simulink model "Red_problema1_imc_nuevo"  (R2021a)
settings: Solver=ode15s  StartTime=0.0  StopTime=500  MinStep=2e-4  RelTol=1e-3
values from neighbouring files (symbols this model uses):
  area1 = 35.35580060269119    (= 35.3558006027)    [INI.m]    (also in INI_identify.m)
  area1_ini = 34.71685026942442    (= 34.7168502694)    [INI.m]    (also in INI_identify.m)
  area2 = 44.26996515041091    (= 44.2699651504)    [INI.m]    (also in INI_identify.m)
  area2_ini = 42.266246191143715    (= 42.2662461911)    [INI.m]    (also in INI_identify.m)
  area3 = 23.697558590692203    (= 23.6975585907)    [INI.m]    (also in INI_identify.m)
  area3_ini = 22.769214035906693    (= 22.7692140359)    [INI.m]    (also in INI_identify.m)
  area4 = 2.513764303269934    (= 2.51376430327)    [INI.m]    (also in INI_identify.m)
  area4_ini = 2.513764303269934    (= 2.51376430327)    [INI.m]    (also in INI_identify.m)
  area_time = 0    [INI.m]    (also in INI_identify.m)
  bypass_time = 50    [INI.m]    (also in INI_identify.m)
  d_time = 50    [INI.m]    (also in INI_identify.m)
  fcin1 = 0    [INI.m]    (also in INI_identify.m; script_variar_vms.m)
  fcin2 = 0    [INI.m]    (also in INI_identify.m; script_variar_vms.m)
  fcu = 0    [INI.m]    (also in INI_identify.m; script_variar_vms.m)
  fcu_time = 50    [INI.m]    (also in INI_identify.m)
  fhin1 = 0    [INI.m]    (also in INI_identify.m; script_variar_vms.m)
  fhin2 = 0    [INI.m]    (also in INI_identify.m; script_variar_vms.m)
  initials = [uh112_initial uh211_initial uh222_initial uc112_initial uc211_initial uc222_initial fcu_initial]    [INI.m]    (also in INI_identify.m)
  tcin1 = 0    [INI.m]    (also in INI_identify.m; pert_max.m = -5; script_variar_vms.m)
  tcin2 = 0    [INI.m]    (also in INI_identify.m; pert_max.m = -5; script_variar_vms.m)
  thin1 = 0    [INI.m]    (also in INI_identify.m; pert_max.m = 5; script_variar_vms.m)
  thin2 = 0    [INI.m]    (also in INI_identify.m; script_variar_vms.m)
  uc112 = 0.0    (= 0)    [INI.m]    (also in INI_identify.m; script_variar_vms.m)
  uc112_initial = uc112    (= 0)    [INI.m]    (also in INI_identify.m)
  uc211 = 0.0    (= 0)    [INI.m]    (also in INI_identify.m; script_variar_vms.m)
  uc211_initial = uc211    (= 0)    [INI.m]    (also in INI_identify.m)
  uc222 = 0.0    (= 0)    [INI.m]    (also in INI_identify.m; script_variar_vms.m)
  uc222_initial = uc222    (= 0)    [INI.m]    (also in INI_identify.m)
  uh112 = 0.014935258720777856    (= 0.0149352587208)    [INI.m]    (also in INI_identify.m; script_variar_vms.m)
  uh112_initial = uh112    (= 0.0149352587208)    [INI.m]    (also in INI_identify.m)
  uh211 = 0.05299733469368127    (= 0.0529973346937)    [INI.m]    (also in INI_identify.m; script_variar_vms.m)
  uh211_initial = uh211    (= 0.0529973346937)    [INI.m]    (also in INI_identify.m)
  uh222 = 0.08194236649754925    (= 0.0819423664975)    [INI.m]    (also in INI_identify.m; script_variar_vms.m)
  uh222_initial = uh222    (= 0.0819423664975)    [INI.m]    (also in INI_identify.m)
libraries: simulink x4, cstblocks x2
settings Model: Creator=fzpat  LastModifiedBy=LENOVO_T14
settings DataIOCC: SaveFinalState=on  SaveFormat=Array  SaveState=on
settings DebuggingCC: AlgebraicLoopMsg=none  ArtificialAlgebraicLoopMsg=none

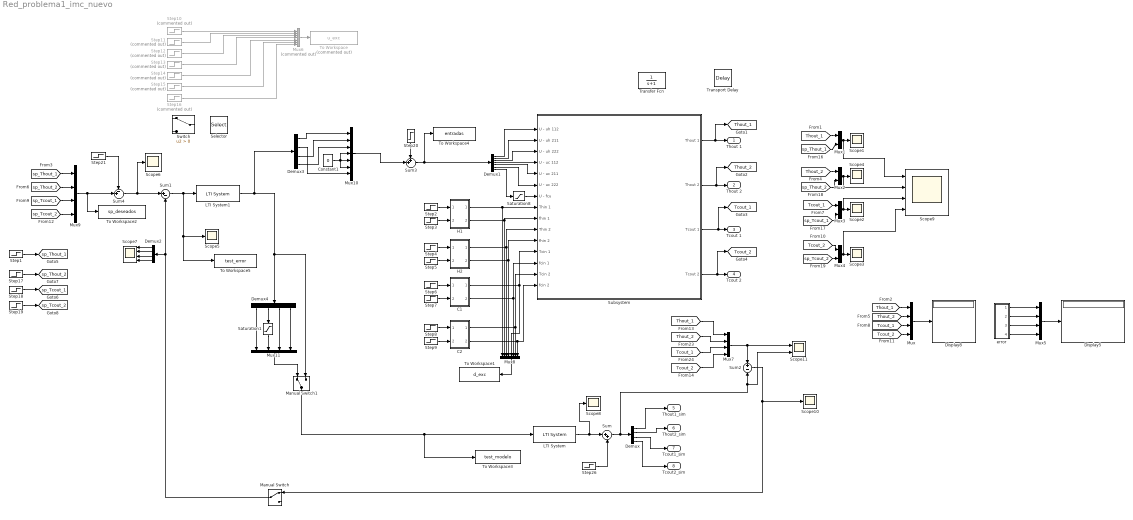
== system Red_problema1_imc_nuevo ==
  C1 : Subsystem
  "C2 " : Subsystem
  Constant1 : Constant  Value=0
  Demux{,2..4} (4 alike) : Demux
  Demux1 : Demux  Outputs=7
  Display5 : Display
  Display8 : Display
  "H1 " : Subsystem
  H2 : Subsystem
  LTI System : cstblocks/LTI System  sys=Gvn1  IC=[]
  LTI System1 : cstblocks/LTI System  sys=Kimc1  IC=[]
  Manual Switch : ManualSwitch
  Manual Switch1 : ManualSwitch
  Mux{,5,7,9,11} (5 alike) : Mux
  Mux{1..4} (4 alike) : Mux  Inputs=2
  Mux10 : Mux  Inputs=7
  Mux6 : Mux  Commented=on  Inputs=7
  Mux8 : Mux  Inputs=8
  Saturation1 : Saturate  UpperLimit=-1e-9  LowerLimit=-29.95
  Saturation8 : Saturate  UpperLimit=-1e-9  LowerLimit=-29.95
  Scope{1..6,8,10} (8 alike) : Scope
  Scope11 : Scope  NumInputPorts=2
  Scope7 : Scope  NumInputPorts=4
  Scope9 : Scope  NumInputPorts=4
  Selector : Selector  InputPortWidth=3  IndexOptions=Index vector (port)  Indices=[1 3]  OutputSizes=1
  Step1 : Step  Time=1e9  Before=385  After=385
  Step10 : Step  Commented=on  Time=bypass_time  Before=uh112_initial  After=uh112
  Step11 : Step  Commented=on  Time=bypass_time  Before=uh211_initial  After=uh211
  Step12 : Step  Commented=on  Time=bypass_time  Before=uh222_initial  After=uh222
  Step13 : Step  Commented=on  Time=bypass_time  Before=uc112_initial  After=uc112
  Step14 : Step  Commented=on  Time=bypass_time  Before=uc211_initial  After=uc211
  Step15 : Step  Commented=on  Time=bypass_time  Before=uc222_initial  After=uc222
  Step16 : Step  Commented=on  Time=fcu_time  After=fcu
  Step17 : Step  Time=1e10  Before=400  After=400
  Step18 : Step  Time=1e9  Before=560  After=560
  Step19 : Step  Time=1e10  Before=340  After=340
  Step2 : Step  Time=d_time  After=thin1
  Step20 : Step  Time=0  Before=initials  After=initials
  Step21 : Step  Time=0  Before=setpoints'  After=setpoints'
  Step26 : Step  Time=0  Before=setpoints'  After=setpoints'
  Step3 : Step  Time=d_time  After=fhin1
  Step4 : Step  Time=d_time  After=thin2
  Step5 : Step  Time=d_time  After=fhin2
  Step6 : Step  Time=d_time  After=tcin1
  Step7 : Step  Time=d_time  After=fcin1
  Step8 : Step  Time=d_time  After=tcin2
  Step9 : Step  Time=d_time  After=fcin2
  Subsystem : Subsystem  TreatAsAtomicUnit=on
      settings: MinAlgLoopOccurrences=on
  Sum : Sum  Inputs=|++
  Sum1 : Sum  Inputs=|+-
  Sum2 : Sum  Inputs=+-
  Sum3 : Sum  Inputs=++|
  Sum4 : Sum  Inputs=-+|
  Switch : Switch  Criteria=u2 > Threshold
  To Workspace : ToWorkspace  Commented=on  VariableName=u_exc  SampleTime=-1
  To Workspace1 : ToWorkspace  VariableName=d_exc  SampleTime=-1
  To Workspace2 : ToWorkspace  VariableName=sp_deseados  SampleTime=-1
  To Workspace3 : ToWorkspace  VariableName=test_modelo  SampleTime=-1
  To Workspace4 : ToWorkspace  VariableName=entradas  SampleTime=-1
  To Workspace5 : ToWorkspace  VariableName=test_error  SampleTime=-1
  Transfer Fcn : TransferFcn  Denominator=[1 1]
  Transport Delay : TransportDelay
  error : Subsystem
  Thout 1 : Outport  VectorParamsAs1DForOutWhenUnconnected=off
  Thout 2 : Outport  Port=2  VectorParamsAs1DForOutWhenUnconnected=off
  Tcout 1 : Outport  Port=3  VectorParamsAs1DForOutWhenUnconnected=off
  Tcout 2 : Outport  Port=4  VectorParamsAs1DForOutWhenUnconnected=off
  Thout1_sim : Outport  Port=5  VectorParamsAs1DForOutWhenUnconnected=off
  Thout2_sim : Outport  Port=6  VectorParamsAs1DForOutWhenUnconnected=off
  Tcout1_sim : Outport  Port=7  VectorParamsAs1DForOutWhenUnconnected=off
  Tcout2_sim : Outport  Port=8  VectorParamsAs1DForOutWhenUnconnected=off
  tag scope: Tcout_1=global, Tcout_2=global, Thout_1=global, Thout_2=global, sp_Tcout_1=global, sp_Tcout_2=global, sp_Thout_1=global, sp_Thout_2=global
  wires:
  Step4/1 -> H2/1(Thin 2)
  Mux5/1 -> Display5/1
  [sp_Tcout_2] -> Mux4/2
  Step16/1 -> Mux6/7
  [Tcout_1] -> Mux/3
  Step15/1 -> Mux6/6
  [Thout_1] -> Mux/1
  error/1(Out1) -> Mux5/1
  [Tcout_1] -> Mux3/1
  Step1/1 -> [sp_Thout_1]
  [Thout_1] -> Mux1/1
  [Tcout_2] -> Mux/4
  Step8/1 -> "C2 "/1(Tcin 2)
  C1/1(Out1) -> Subsystem/12(Tcin 1), Mux8/5
  "C2 "/2(Out2) -> Subsystem/15(fcin 2), Mux8/8
  "C2 "/1(Out1) -> Subsystem/14(Tcin 2), Mux8/7
  C1/2(Out2) -> Subsystem/13(fcin 1), Mux8/6
  Subsystem/4(Tcout 2) -> [Tcout_2], Tcout 2/1
  Step7/1 -> C1/2(fcin 1)
  H2/1(Out1) -> Subsystem/10(Thin 2), Mux8/3
  H2/2(Out2) -> Subsystem/11(fhin 2), Mux8/4
  "H1 "/2(Out2) -> Subsystem/9(fhin 1), Mux8/2
  Step10/1 -> Mux6/1
  Subsystem/1(Thout 1) -> [Thout_1], Thout 1/1
  Step9/1 -> "C2 "/2(fcin 2)
  Subsystem/3(Tcout 1) -> Tcout 1/1, [Tcout_1]
  [Thout_2] -> Mux/2
  LTI System/1 -> Scope8/1, Sum/1
  Step26/1 -> Sum/2
  Demux/2 -> Thout2_sim/1
  "H1 "/1(Out1) -> Mux8/1, Subsystem/8(Thin 1)
  Sum/1 -> Scope11/2, Sum2/2, Demux/1
  Step19/1 -> [sp_Tcout_2]
  Step14/1 -> Mux6/5
  Mux3/1 -> Scope9/3, Scope2/1
  Demux/1 -> Thout1_sim/1
  Step18/1 -> [sp_Tcout_1]
  error/4(Out4) -> Mux5/4
  [Tcout_2] -> Mux4/1
  Mux1/1 -> Scope9/1, Scope1/1
  Demux/4 -> Tcout2_sim/1
  Step13/1 -> Mux6/4
  Demux/3 -> Tcout1_sim/1
  Step12/1 -> Mux6/3
  Step17/1 -> [sp_Thout_2]
  [Thout_2] -> Mux2/1
  Mux2/1 -> Scope9/2, Scope4/1
  Mux8/1 -> To Workspace1/1
  [sp_Tcout_1] -> Mux3/2
  error/3(Out3) -> Mux5/3
  Step6/1 -> C1/1(Tcin 1)
  [sp_Thout_1] -> Mux1/2
  Mux4/1 -> Scope9/4, Scope3/1
  Step11/1 -> Mux6/2
  [sp_Thout_2] -> Mux2/2
  Mux6/1 -> To Workspace/1
  Subsystem/2(Thout 2) -> [Thout_2], Thout 2/1
  error/2(Out2) -> Mux5/2
  Step5/1 -> H2/2(fhin 2)
  Mux/1 -> Display8/1
  Step3/1 -> "H1 "/2(fhin 1)
  Demux1/1 -> Subsystem/1(U - uh 112)
  Demux1/2 -> Subsystem/2(U - uh 211)
  Demux1/3 -> Subsystem/3(U - uh 222)
  Demux1/4 -> Subsystem/4(U - uc 112)
  Demux1/5 -> Subsystem/5(U - uc 211)
  Demux1/6 -> Subsystem/6(U - uc 222)
  [sp_Thout_1] -> Mux9/1
  [sp_Thout_2] -> Mux9/2
  [sp_Tcout_2] -> Mux9/4
  [sp_Tcout_1] -> Mux9/3
  Mux9/1 -> Sum4/2, To Workspace2/1
  Sum1/1 -> To Workspace5/1, Scope5/1, LTI System1/1
  Mux7/1 -> Sum2/1, Scope11/1
  [Thout_1] -> Mux7/1
  [Thout_2] -> Mux7/2
  [Tcout_1] -> Mux7/3
  [Tcout_2] -> Mux7/4
  Demux1/7 -> Saturation8/1
  Sum3/1 -> Demux1/1, To Workspace4/1
  Manual Switch/1 -> Demux2/1, Sum1/2
  LTI System1/1 -> Manual Switch1/2, Demux4/1, Demux3/1
  Sum2/1 -> Manual Switch/1, Scope10/1
  Demux2/1 -> Scope7/1
  Demux2/2 -> Scope7/2
  Demux2/3 -> Scope7/3
  Demux2/4 -> Scope7/4
  Demux3/1 -> Mux10/1
  Demux3/2 -> Mux10/7
  Demux3/3 -> Mux10/2
  Demux3/4 -> Mux10/3
  Constant1/1 -> Mux10/6, Mux10/4, Mux10/5
  Step21/1 -> Sum4/1
  Sum4/1 -> Scope6/1, Sum1/1
  Step20/1 -> Sum3/1
  Mux10/1 -> Sum3/2
  Step2/1 -> "H1 "/1(Thin 1)
  Saturation8/1 -> Subsystem/7(U - fcu)
  Mux11/1 -> Manual Switch1/1
  Demux4/2 -> Saturation1/1
  Saturation1/1 -> Mux11/2
  Demux4/1 -> Mux11/1
  Demux4/3 -> Mux11/3
  Demux4/4 -> Mux11/4
  Manual Switch1/1 -> LTI System/1, To Workspace3/1

== system Red_problema1_imc_nuevo/C1 ==
  Tcin 1 : Inport
  fcin 1 : Inport  Port=2
  Add2 : Sum
  Add3 : Sum
  Constant3 : Constant  Value=300
  Constant4 : Constant  Value=20
  Out1 : Outport  VectorParamsAs1DForOutWhenUnconnected=off
  Out2 : Outport  Port=2  VectorParamsAs1DForOutWhenUnconnected=off
  wires:
  Constant3/1 -> Add2/1
  Constant4/1 -> Add3/1
  Tcin 1/1 -> Add2/2
  fcin 1/1 -> Add3/2
  Add2/1 -> Out1/1
  Add3/1 -> Out2/1

== system Red_problema1_imc_nuevo/C2  ==
  Tcin 2 : Inport
  fcin 2 : Inport  Port=2
  Add4 : Sum
  Add5 : Sum
  Constant5 : Constant  Value=280
  Constant6 : Constant  Value=30
  Out1 : Outport  VectorParamsAs1DForOutWhenUnconnected=off
  Out2 : Outport  Port=2  VectorParamsAs1DForOutWhenUnconnected=off
  wires:
  Constant5/1 -> Add4/1
  Constant6/1 -> Add5/1
  Tcin 2/1 -> Add4/2
  fcin 2/1 -> Add5/2
  Add4/1 -> Out1/1
  Add5/1 -> Out2/1

== system Red_problema1_imc_nuevo/H1  ==
  Thin 1 : Inport
  fhin 1 : Inport  Port=2
  Add : Sum
  Add1 : Sum
  Constant1 : Constant  Value=620
  Constant2 : Constant  Value=10
  Out1 : Outport  VectorParamsAs1DForOutWhenUnconnected=off
  Out2 : Outport  Port=2  VectorParamsAs1DForOutWhenUnconnected=off
  wires:
  Constant1/1 -> Add/1
  Thin 1/1 -> Add/2
  Add/1 -> Out1/1
  Constant2/1 -> Add1/1
  fhin 1/1 -> Add1/2
  Add1/1 -> Out2/1

== system Red_problema1_imc_nuevo/H2 ==
  Thin 2 : Inport
  fhin 2 : Inport  Port=2
  Add : Sum
  Add1 : Sum
  Constant1 : Constant  Value=720
  Constant2 : Constant  Value=15
  Out1 : Outport  VectorParamsAs1DForOutWhenUnconnected=off
  Out2 : Outport  Port=2  VectorParamsAs1DForOutWhenUnconnected=off
  wires:
  Constant1/1 -> Add/1
  Thin 2/1 -> Add/2
  Add/1 -> Out1/1
  Constant2/1 -> Add1/1
  fhin 2/1 -> Add1/2
  Add1/1 -> Out2/1

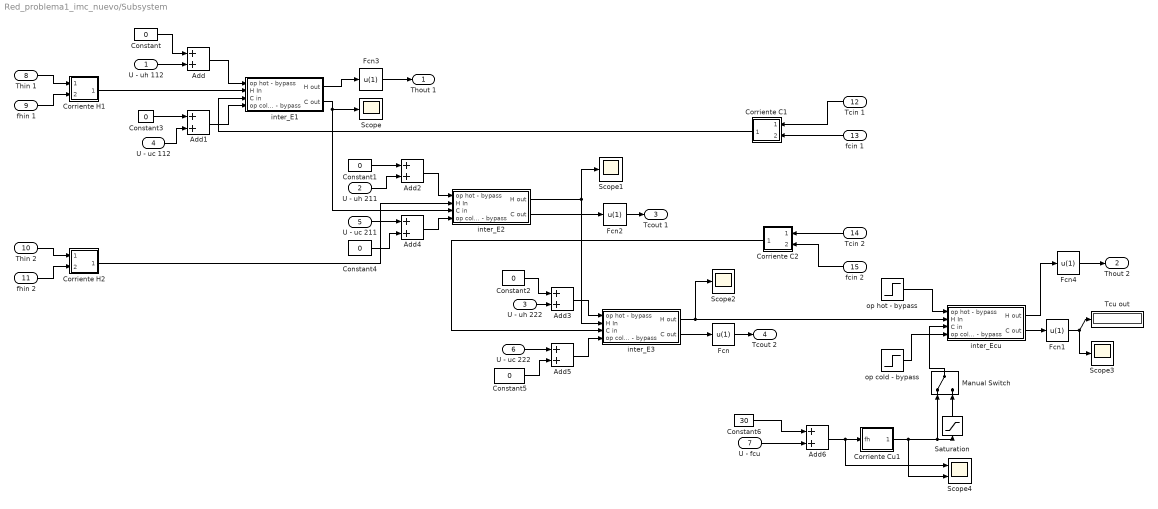
== system Red_problema1_imc_nuevo/Subsystem ==
  U - uh 112 : Inport
  U - uh 211 : Inport  Port=2
  U - uh 222 : Inport  Port=3
  U - uc 112 : Inport  Port=4
  U - uc 211 : Inport  Port=5
  U - uc 222 : Inport  Port=6
  U - fcu : Inport  Port=7
  Thin 1 : Inport  Port=8
  fhin 1 : Inport  Port=9
  Thin 2 : Inport  Port=10
  fhin 2 : Inport  Port=11
  Tcin 1 : Inport  Port=12
  fcin 1 : Inport  Port=13
  Tcin 2 : Inport  Port=14
  fcin 2 : Inport  Port=15
  Add{,1..6} (7 alike) : Sum
  Constant{,1..5} (6 alike) : Constant  Value=0
  Constant6 : Constant  Value=30
  Corriente C1 : Subsystem
  Corriente C2 : Subsystem
  Corriente Cu1 : Subsystem
  Corriente H1 : Subsystem
  Corriente H2 : Subsystem
  Fcn{,1..4} (5 alike) : Fcn  Expr=u(1)
  Manual Switch : ManualSwitch
  Saturation : Saturate  UpperLimit=inf  LowerLimit=1e-9
  Scope{,1..3} (4 alike) : Scope
  Scope4 : Scope  NumInputPorts=2
  Tcu out : Display
  inter_E1 : Subsystem
  inter_E2 : Subsystem
  inter_E3 : Subsystem
  inter_Ecu : Subsystem
  op cold - bypass : Step  Time=0  After=0  SampleTime=0
  op hot - bypass : Step  Time=0  After=0  SampleTime=0
  Thout 1 : Outport  VectorParamsAs1DForOutWhenUnconnected=off
  Thout 2 : Outport  Port=2  VectorParamsAs1DForOutWhenUnconnected=off
  Tcout 1 : Outport  Port=3  VectorParamsAs1DForOutWhenUnconnected=off
  Tcout 2 : Outport  Port=4  VectorParamsAs1DForOutWhenUnconnected=off
  wires:
  inter_Ecu/2(C out) -> Fcn1/1
  op cold - bypass/1 -> inter_Ecu/4("op cold - bypass ")
  Corriente Cu1/1(Out1) -> Saturation/1, Manual Switch/1, Scope4/2
  Corriente H1/1(Out1) -> inter_E1/2(H In)
  inter_Ecu/1(H out) -> Fcn4/1
  Fcn1/1 -> Scope3/1, Tcu out/1
  op hot - bypass/1 -> inter_Ecu/1("op hot - bypass ")
  Thin 1/1 -> Corriente H1/1(In1)
  fhin 1/1 -> Corriente H1/2(In2)
  Tcin 1/1 -> Corriente C1/1(In1)
  fcin 1/1 -> Corriente C1/2(In2)
  Tcin 2/1 -> Corriente C2/1(In1)
  fcin 2/1 -> Corriente C2/2(In2)
  U - uh 112/1 -> Add/2
  Constant/1 -> Add/1
  U - uc 112/1 -> Add1/2
  Add1/1 -> inter_E1/4("op cold - bypass ")
  Add/1 -> inter_E1/1("op hot - bypass ")
  U - uh 211/1 -> Add2/2
  Constant1/1 -> Add2/1
  Add2/1 -> inter_E2/1("op hot - bypass ")
  U - uh 222/1 -> Add3/2
  Add3/1 -> inter_E3/1("op hot - bypass ")
  Constant2/1 -> Add3/1
  Constant3/1 -> Add1/1
  U - uc 211/1 -> Add4/1
  Constant4/1 -> Add4/2
  Add4/1 -> inter_E2/4("op cold - bypass ")
  U - uc 222/1 -> Add5/1
  Constant5/1 -> Add5/2
  Add5/1 -> inter_E3/4("op cold - bypass ")
  Add6/1 -> Scope4/1, Corriente Cu1/1(fh)
  Constant6/1 -> Add6/1
  Thin 2/1 -> Corriente H2/1(In1)
  fhin 2/1 -> Corriente H2/2(In2)
  Corriente H2/1(Out1) -> inter_E2/2(H In)
  Corriente C1/1(Out1) -> inter_E1/3(C in)
  inter_E1/1(H out) -> Fcn3/1
  Fcn3/1 -> Thout 1/1
  inter_E1/2(C out) -> inter_E2/3(C in), Scope/1
  Corriente C2/1(Out1) -> inter_E3/3(C in)
  inter_E3/2(C out) -> Fcn/1
  Fcn/1 -> Tcout 2/1
  inter_E2/1(H out) -> Scope1/1, inter_E3/2(H In)
  inter_E3/1(H out) -> Scope2/1, inter_Ecu/2(H In)
  Fcn4/1 -> Thout 2/1
  inter_E2/2(C out) -> Fcn2/1
  Fcn2/1 -> Tcout 1/1
  U - fcu/1 -> Add6/2
  Saturation/1 -> Manual Switch/2
  Manual Switch/1 -> inter_Ecu/3(C in)

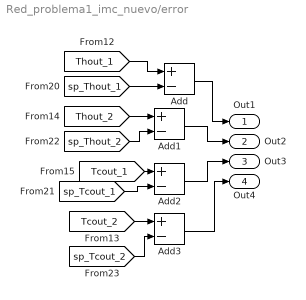
== system Red_problema1_imc_nuevo/error ==
  Add{,1..3} (4 alike) : Sum  Inputs=+-
  Out1 : Outport  VectorParamsAs1DForOutWhenUnconnected=off
  Out2 : Outport  Port=2  VectorParamsAs1DForOutWhenUnconnected=off
  Out3 : Outport  Port=3  VectorParamsAs1DForOutWhenUnconnected=off
  Out4 : Outport  Port=4  VectorParamsAs1DForOutWhenUnconnected=off
  wires:
  [sp_Thout_2] -> Add1/2
  [sp_Tcout_2] -> Add3/2
  [sp_Tcout_1] -> Add2/2
  [sp_Thout_1] -> Add/2
  [Thout_2] -> Add1/1
  [Thout_1] -> Add/1
  [Tcout_1] -> Add2/1
  [Tcout_2] -> Add3/1
  Add1/1 -> Out2/1
  Add/1 -> Out1/1
  Add3/1 -> Out4/1
  Add2/1 -> Out3/1

== system Red_problema1_imc_nuevo/Subsystem/Corriente C1 ==
  In1 : Inport
  In2 : Inport  Port=2
  Mux5 : Mux  Inputs=3
  Terminator : Terminator
  Terminator1 : Terminator
  fc : Step  Before=13  After=13  SampleTime=0
  hc : Step  Before=1  SampleTime=0
  tc : Step  Before=333  After=333  SampleTime=0
  Out1 : Outport  VectorParamsAs1DForOutWhenUnconnected=off
  wires:
  Mux5/1 -> Out1/1
  hc/1 -> Mux5/3
  In1/1 -> Mux5/1
  In2/1 -> Mux5/2
  fc/1 -> Terminator/1
  tc/1 -> Terminator1/1

== system Red_problema1_imc_nuevo/Subsystem/Corriente C2 ==
  In1 : Inport
  In2 : Inport  Port=2
  Mux5 : Mux  Inputs=3
  Terminator : Terminator
  Terminator1 : Terminator
  fh : Step  Before=12  After=12  SampleTime=0
  hh : Step  Before=1  SampleTime=0
  th : Step  Time=2  Before=293  After=293  SampleTime=0
  Out1 : Outport  VectorParamsAs1DForOutWhenUnconnected=off
  wires:
  hh/1 -> Mux5/3
  Mux5/1 -> Out1/1
  In1/1 -> Mux5/1
  In2/1 -> Mux5/2
  fh/1 -> Terminator/1
  th/1 -> Terminator1/1

== system Red_problema1_imc_nuevo/Subsystem/Corriente Cu1 ==
  fh : Inport
  Mux5 : Mux  Inputs=3
  hh : Step  Before=1  SampleTime=0
  th : Step  Time=2  Before=283  After=283  SampleTime=0
  Out1 : Outport  VectorParamsAs1DForOutWhenUnconnected=off
  wires:
  hh/1 -> Mux5/3
  th/1 -> Mux5/1
  Mux5/1 -> Out1/1
  fh/1 -> Mux5/2

== system Red_problema1_imc_nuevo/Subsystem/Corriente H1 ==
  In1 : Inport
  In2 : Inport  Port=2
  Mux5 : Mux  Inputs=3
  Terminator : Terminator
  Terminator1 : Terminator
  fh : Step  Before=20  After=20  SampleTime=0
  hh : Step  Before=1  SampleTime=0
  th : Step  Time=2  Before=423  After=423  SampleTime=0
  Out1 : Outport  VectorParamsAs1DForOutWhenUnconnected=off
  wires:
  Mux5/1 -> Out1/1
  hh/1 -> Mux5/3
  In1/1 -> Mux5/1
  In2/1 -> Mux5/2
  th/1 -> Terminator/1
  fh/1 -> Terminator1/1

== system Red_problema1_imc_nuevo/Subsystem/Corriente H2 ==
  In1 : Inport
  In2 : Inport  Port=2
  Mux5 : Mux  Inputs=3
  Terminator : Terminator
  Terminator1 : Terminator
  fh : Step  Before=20  After=20  SampleTime=0
  hh : Step  Before=1  SampleTime=0
  th : Step  Time=2  Before=423  After=423  SampleTime=0
  Out1 : Outport  VectorParamsAs1DForOutWhenUnconnected=off
  wires:
  Mux5/1 -> Out1/1
  hh/1 -> Mux5/3
  In1/1 -> Mux5/1
  In2/1 -> Mux5/2
  th/1 -> Terminator/1
  fh/1 -> Terminator1/1

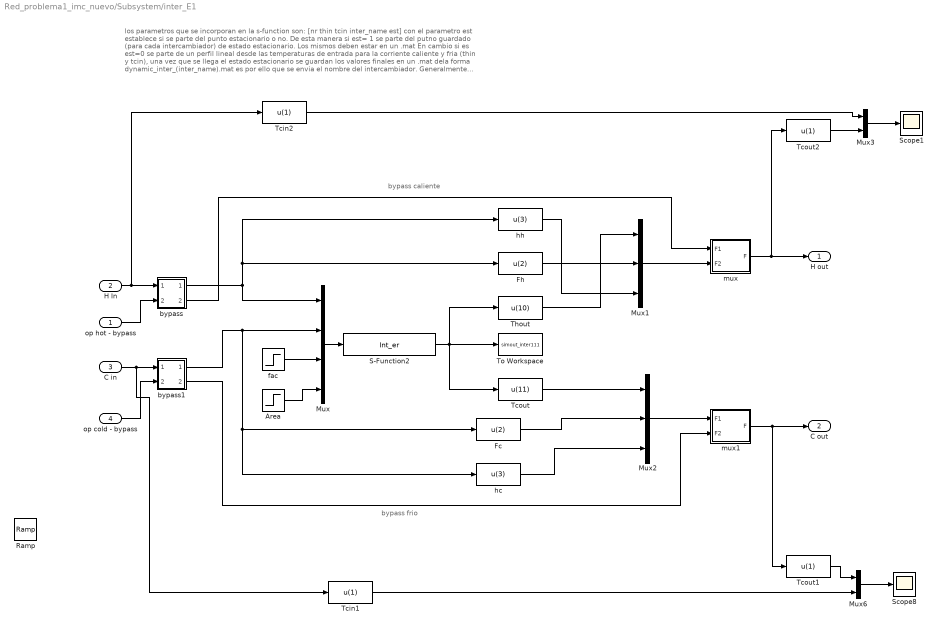
== system Red_problema1_imc_nuevo/Subsystem/inter_E1 ==
  note: los parametros que se incorporan en la s-function son: [nr thin tcin inter_name est]
      | con el parametro est establece si se parte del punto estacionario o no. De esta manera si est= 1 se parte del putno guardado (para cada intercambiador) de estado estacionario. Los mismos deben estar en un .mat
      | En cambio si es est=0 se parte de un perfil lineal  desde las temperaturas de entrada para la corriente caliente y fria (thin y tcin), una vez que se llega el estado estacionario se guardan los valores finales en un .mat
      | dela forma dynamic_inter_(inter_name).mat   es por ello que se envia el nombre del intercambiador.
      | Generalmente para la primera vez que se corre la red se una est=0 para que llegue al estado estacionario y una vez que se alcanzó se vuelve a correr con est= 1 para hacer análisis de control
  note: bypass frio
  note: bypass caliente
  "op hot - bypass " : Inport
  H In : Inport  Port=2
  C in : Inport  Port=3
  "op cold - bypass " : Inport  Port=4
  Area : Step  Time=area_time  Before=area1_ini  After=area1  SampleTime=0
  Fc : Fcn  Expr=u(2)
  Fh : Fcn  Expr=u(2)
  Mux : Mux
  Mux1 : Mux  Inputs=3
  Mux2 : Mux  Inputs=3
  Mux3 : Mux  Inputs=2
  Mux6 : Mux  Inputs=2
  Ramp : simulink/Sources/Ramp  slope=0  start=0  InitialOutput=0
  S-Function2 : S-Function  FunctionName=Int_er  Parameters=10 620 300 112 2  SFunctionDeploymentMode=off  EnableBusSupport=off
  Scope1 : Scope
  Scope8 : Scope
  Tcin1 : Fcn  Expr=u(1)
  Tcin2 : Fcn  Expr=u(1)
  Tcout : Fcn  Expr=u(11)
  Tcout1 : Fcn  Expr=u(1)
  Tcout2 : Fcn  Expr=u(1)
  Thout : Fcn  Expr=u(10)
  To Workspace : ToWorkspace  VariableName=simout_inter111  SampleTime=-1
  bypass : Subsystem
  bypass1 : Subsystem
  fac : Step  After=0  SampleTime=0
  hc : Fcn  Expr=u(3)
  hh : Fcn  Expr=u(3)
  mux : Subsystem
  mux1 : Subsystem
  H out : Outport  VectorParamsAs1DForOutWhenUnconnected=off
  C out : Outport  Port=2  VectorParamsAs1DForOutWhenUnconnected=off
  wires:
  Tcout/1 -> Mux2/1
  Thout/1 -> Mux1/1
  Fc/1 -> Mux2/2
  Fh/1 -> Mux1/2
  S-Function2/1 -> Thout/1, To Workspace/1, Tcout/1
  Mux/1 -> S-Function2/1
  fac/1 -> Mux/3
  hc/1 -> Mux2/3
  hh/1 -> Mux1/3
  Area/1 -> Mux/4
  H In/1 -> Tcin2/1, bypass/1(1)
  bypass/1(" 1") -> Mux/1, Fh/1, hh/1
  Mux1/1 -> mux/2(F2)
  bypass/2(" 2") -> mux/1(F1)
  "op hot - bypass "/1 -> bypass/2(u122)
  C in/1 -> Tcin1/1, bypass1/1(1)
  "op cold - bypass "/1 -> bypass1/2(u122)
  mux/1("F ") -> Tcout2/1, H out/1
  Mux2/1 -> mux1/1(F1)
  mux1/1("F ") -> Tcout1/1, C out/1
  bypass1/1(" 1") -> hc/1, Fc/1, Mux/2
  bypass1/2(" 2") -> mux1/2(F2)
  Mux6/1 -> Scope8/1
  Tcout1/1 -> Mux6/1
  Tcin1/1 -> Mux6/2
  Mux3/1 -> Scope1/1
  Tcout2/1 -> Mux3/2
  Tcin2/1 -> Mux3/1

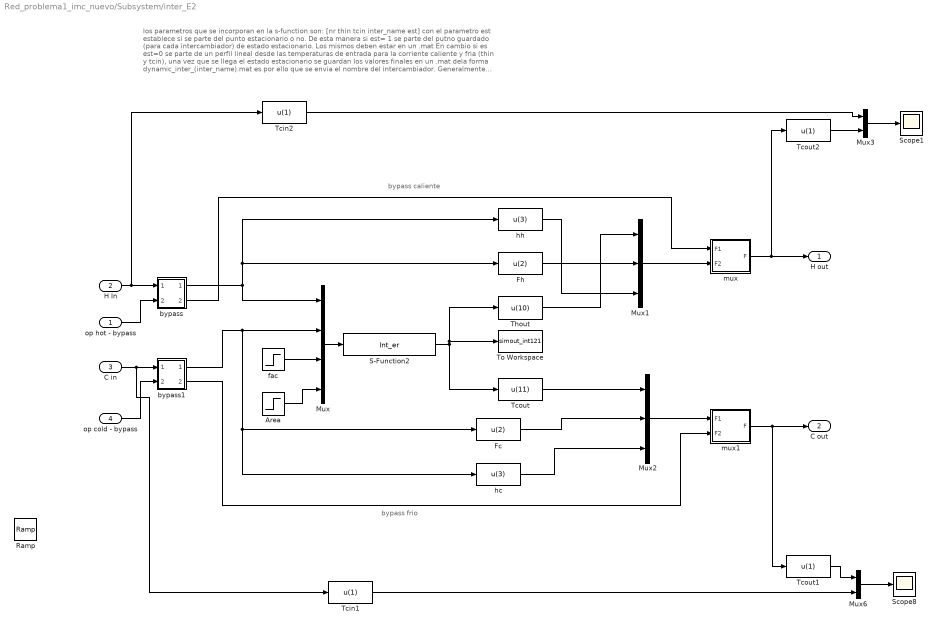
== system Red_problema1_imc_nuevo/Subsystem/inter_E2 ==
  note: bypass caliente
  note: bypass frio
  note: los parametros que se incorporan en la s-function son: [nr thin tcin inter_name est]
      | con el parametro est establece si se parte del punto estacionario o no. De esta manera si est= 1 se parte del putno guardado (para cada intercambiador) de estado estacionario. Los mismos deben estar en un .mat
      | En cambio si es est=0 se parte de un perfil lineal  desde las temperaturas de entrada para la corriente caliente y fria (thin y tcin), una vez que se llega el estado estacionario se guardan los valores finales en un .mat
      | dela forma dynamic_inter_(inter_name).mat   es por ello que se envia el nombre del intercambiador.
      | Generalmente para la primera vez que se corre la red se una est=0 para que llegue al estado estacionario y una vez que se alcanzó se vuelve a correr con est= 1 para hacer análisis de control
  "op hot - bypass " : Inport
  H In : Inport  Port=2
  C in : Inport  Port=3
  "op cold - bypass " : Inport  Port=4
  Area : Step  Time=area_time  Before=area2_ini  After=area2  SampleTime=0
  Fc : Fcn  Expr=u(2)
  Fh : Fcn  Expr=u(2)
  Mux : Mux
  Mux1 : Mux  Inputs=3
  Mux2 : Mux  Inputs=3
  Mux3 : Mux  Inputs=2
  Mux6 : Mux  Inputs=2
  Ramp : simulink/Sources/Ramp  slope=0  start=0  InitialOutput=0
  S-Function2 : S-Function  FunctionName=Int_er  Parameters=10 720 417.5 211 2  SFunctionDeploymentMode=off  EnableBusSupport=off
  Scope1 : Scope
  Scope8 : Scope
  Tcin1 : Fcn  Expr=u(1)
  Tcin2 : Fcn  Expr=u(1)
  Tcout : Fcn  Expr=u(11)
  Tcout1 : Fcn  Expr=u(1)
  Tcout2 : Fcn  Expr=u(1)
  Thout : Fcn  Expr=u(10)
  To Workspace : ToWorkspace  VariableName=simout_int121  SampleTime=-1
  bypass : Subsystem
  bypass1 : Subsystem
  fac : Step  After=0  SampleTime=0
  hc : Fcn  Expr=u(3)
  hh : Fcn  Expr=u(3)
  mux : Subsystem
  mux1 : Subsystem
  H out : Outport  VectorParamsAs1DForOutWhenUnconnected=off
  C out : Outport  Port=2  VectorParamsAs1DForOutWhenUnconnected=off
  wires:
  Tcin2/1 -> Mux3/1
  Tcout2/1 -> Mux3/2
  Mux3/1 -> Scope1/1
  Tcin1/1 -> Mux6/2
  Tcout1/1 -> Mux6/1
  Mux6/1 -> Scope8/1
  bypass1/2(" 2") -> mux1/2(F2)
  bypass1/1(" 1") -> Mux/2, Fc/1, hc/1
  mux1/1("F ") -> C out/1, Tcout1/1
  Mux2/1 -> mux1/1(F1)
  mux/1("F ") -> H out/1, Tcout2/1
  "op cold - bypass "/1 -> bypass1/2(u122)
  C in/1 -> bypass1/1(1), Tcin1/1
  "op hot - bypass "/1 -> bypass/2(u122)
  bypass/2(" 2") -> mux/1(F1)
  Mux1/1 -> mux/2(F2)
  bypass/1(" 1") -> hh/1, Fh/1, Mux/1
  H In/1 -> bypass/1(1), Tcin2/1
  Area/1 -> Mux/4
  hh/1 -> Mux1/3
  hc/1 -> Mux2/3
  fac/1 -> Mux/3
  Mux/1 -> S-Function2/1
  S-Function2/1 -> Tcout/1, To Workspace/1, Thout/1
  Fh/1 -> Mux1/2
  Fc/1 -> Mux2/2
  Thout/1 -> Mux1/1
  Tcout/1 -> Mux2/1

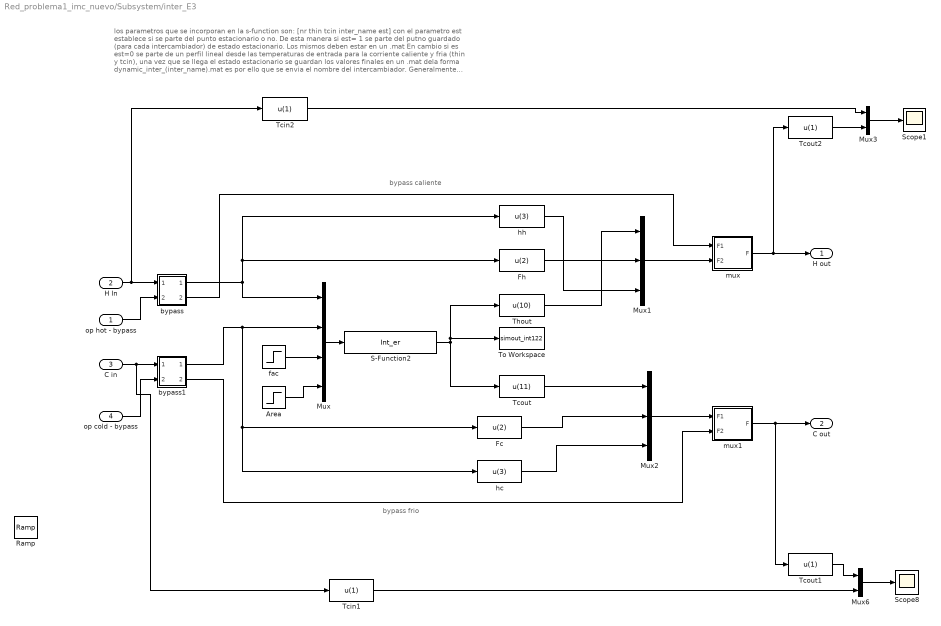
== system Red_problema1_imc_nuevo/Subsystem/inter_E3 ==
  note: bypass frio
  note: bypass caliente
  note: los parametros que se incorporan en la s-function son: [nr thin tcin inter_name est]
      | con el parametro est establece si se parte del punto estacionario o no. De esta manera si est= 1 se parte del putno guardado (para cada intercambiador) de estado estacionario. Los mismos deben estar en un .mat
      | En cambio si es est=0 se parte de un perfil lineal  desde las temperaturas de entrada para la corriente caliente y fria (thin y tcin), una vez que se llega el estado estacionario se guardan los valores finales en un .mat
      | dela forma dynamic_inter_(inter_name).mat   es por ello que se envia el nombre del intercambiador.
      | Generalmente para la primera vez que se corre la red se una est=0 para que llegue al estado estacionario y una vez que se alcanzó se vuelve a correr con est= 1 para hacer análisis de control
  "op hot - bypass " : Inport
  H In : Inport  Port=2
  C in : Inport  Port=3
  "op cold - bypass " : Inport  Port=4
  Area : Step  Time=area_time  Before=area3_ini  After=area3  SampleTime=0
  Fc : Fcn  Expr=u(2)
  Fh : Fcn  Expr=u(2)
  Mux : Mux
  Mux1 : Mux  Inputs=3
  Mux2 : Mux  Inputs=3
  Mux3 : Mux  Inputs=2
  Mux6 : Mux  Inputs=2
  Ramp : simulink/Sources/Ramp  slope=0  start=0  InitialOutput=0
  S-Function2 : S-Function  FunctionName=Int_er  Parameters=10 530 280 222 2  SFunctionDeploymentMode=off  EnableBusSupport=off
  Scope1 : Scope
  Scope8 : Scope
  Tcin1 : Fcn  Expr=u(1)
  Tcin2 : Fcn  Expr=u(1)
  Tcout : Fcn  Expr=u(11)
  Tcout1 : Fcn  Expr=u(1)
  Tcout2 : Fcn  Expr=u(1)
  Thout : Fcn  Expr=u(10)
  To Workspace : ToWorkspace  VariableName=simout_int122  SampleTime=-1
  bypass : Subsystem
  bypass1 : Subsystem
  fac : Step  After=0  SampleTime=0
  hc : Fcn  Expr=u(3)
  hh : Fcn  Expr=u(3)
  mux : Subsystem
  mux1 : Subsystem
  H out : Outport  VectorParamsAs1DForOutWhenUnconnected=off
  C out : Outport  Port=2  VectorParamsAs1DForOutWhenUnconnected=off
  wires:
  Tcout/1 -> Mux2/1
  Thout/1 -> Mux1/1
  Fc/1 -> Mux2/2
  Fh/1 -> Mux1/2
  S-Function2/1 -> Thout/1, To Workspace/1, Tcout/1
  Mux/1 -> S-Function2/1
  fac/1 -> Mux/3
  hc/1 -> Mux2/3
  hh/1 -> Mux1/3
  Area/1 -> Mux/4
  H In/1 -> Tcin2/1, bypass/1(1)
  bypass/1(" 1") -> Mux/1, Fh/1, hh/1
  Mux1/1 -> mux/2(F2)
  bypass/2(" 2") -> mux/1(F1)
  "op hot - bypass "/1 -> bypass/2(u122)
  C in/1 -> Tcin1/1, bypass1/1(1)
  "op cold - bypass "/1 -> bypass1/2(u122)
  mux/1("F ") -> Tcout2/1, H out/1
  Mux2/1 -> mux1/1(F1)
  mux1/1("F ") -> Tcout1/1, C out/1
  bypass1/1(" 1") -> hc/1, Fc/1, Mux/2
  bypass1/2(" 2") -> mux1/2(F2)
  Mux6/1 -> Scope8/1
  Tcout1/1 -> Mux6/1
  Tcin1/1 -> Mux6/2
  Mux3/1 -> Scope1/1
  Tcout2/1 -> Mux3/2
  Tcin2/1 -> Mux3/1

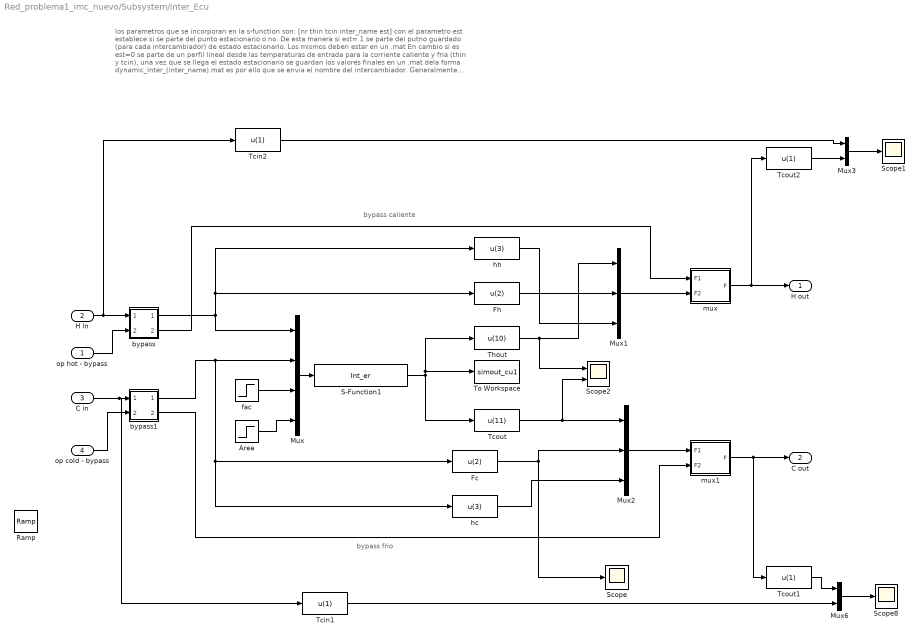
== system Red_problema1_imc_nuevo/Subsystem/inter_Ecu ==
  note: bypass caliente
  note: bypass frio
  note: los parametros que se incorporan en la s-function son: [nr thin tcin inter_name est]
      | con el parametro est establece si se parte del punto estacionario o no. De esta manera si est= 1 se parte del putno guardado (para cada intercambiador) de estado estacionario. Los mismos deben estar en un .mat
      | En cambio si es est=0 se parte de un perfil lineal  desde las temperaturas de entrada para la corriente caliente y fria (thin y tcin), una vez que se llega el estado estacionario se guardan los valores finales en un .mat
      | dela forma dynamic_inter_(inter_name).mat   es por ello que se envia el nombre del intercambiador.
      | Generalmente para la primera vez que se corre la red se una est=0 para que llegue al estado estacionario y una vez que se alcanzó se vuelve a correr con est= 1 para hacer análisis de control
  "op hot - bypass " : Inport
  H In : Inport  Port=2
  C in : Inport  Port=3
  "op cold - bypass " : Inport  Port=4
  Area : Step  Time=area_time  Before=area4_ini  After=area4  SampleTime=0
  Fc : Fcn  Expr=u(2)
  Fh : Fcn  Expr=u(2)
  Mux : Mux
  Mux1 : Mux  Inputs=3
  Mux2 : Mux  Inputs=3
  Mux3 : Mux  Inputs=2
  Mux6 : Mux  Inputs=2
  Ramp : simulink/Sources/Ramp  slope=0.9/150  start=30  InitialOutput=0
  S-Function1 : S-Function  FunctionName=Int_er  Parameters=10 410 293 02 2  SFunctionDeploymentMode=off  EnableBusSupport=off
  Scope : Scope
  Scope1 : Scope
  Scope2 : Scope  NumInputPorts=2
  Scope8 : Scope
  Tcin1 : Fcn  Expr=u(1)
  Tcin2 : Fcn  Expr=u(1)
  Tcout : Fcn  Expr=u(11)
  Tcout1 : Fcn  Expr=u(1)
  Tcout2 : Fcn  Expr=u(1)
  Thout : Fcn  Expr=u(10)
  To Workspace : ToWorkspace  VariableName=simout_cu1  SampleTime=-1
  bypass : Subsystem
  bypass1 : Subsystem
  fac : Step  After=0  SampleTime=0
  hc : Fcn  Expr=u(3)
  hh : Fcn  Expr=u(3)
  mux : Subsystem
  mux1 : Subsystem
  H out : Outport  VectorParamsAs1DForOutWhenUnconnected=off
  C out : Outport  Port=2  VectorParamsAs1DForOutWhenUnconnected=off
  wires:
  Tcin2/1 -> Mux3/1
  Tcout2/1 -> Mux3/2
  Mux3/1 -> Scope1/1
  Tcin1/1 -> Mux6/2
  Tcout1/1 -> Mux6/1
  Mux6/1 -> Scope8/1
  bypass1/2(" 2") -> mux1/2(F2)
  bypass1/1(" 1") -> Mux/2, Fc/1, hc/1
  mux1/1("F ") -> C out/1, Tcout1/1
  Mux2/1 -> mux1/1(F1)
  mux/1("F ") -> H out/1, Tcout2/1
  C in/1 -> bypass1/1(1), Tcin1/1
  "op hot - bypass "/1 -> bypass/2(u122)
  bypass/2(" 2") -> mux/1(F1)
  Mux1/1 -> mux/2(F2)
  bypass/1(" 1") -> hh/1, Fh/1, Mux/1
  H In/1 -> bypass/1(1), Tcin2/1
  Area/1 -> Mux/4
  hh/1 -> Mux1/3
  hc/1 -> Mux2/3
  fac/1 -> Mux/3
  Mux/1 -> S-Function1/1
  S-Function1/1 -> Tcout/1, To Workspace/1, Thout/1
  Fh/1 -> Mux1/2
  Fc/1 -> Mux2/2, Scope/1
  Thout/1 -> Scope2/1, Mux1/1
  Tcout/1 -> Scope2/2, Mux2/1
  "op cold - bypass "/1 -> bypass1/2(u122)

== system Red_problema1_imc_nuevo/Subsystem/inter_E1/bypass ==
  note: la corriete 2 es la corriente del byapass
  note: la corriente 1 es la que se introduce al intercambiador
  1 : Inport
  u122 : Inport  Port=2
  Add : Sum  Inputs=+-
  Manual Switch : ManualSwitch  CurrentSetting=0
  Mux : Mux  Inputs=3
  Mux1 : Mux  Inputs=3
  Product : Product
  Saturation : Saturate  UpperLimit=0.999999999  LowerLimit=0
  T : Fcn  Expr=u(1)
  f : Fcn  Expr=u(2)
  h : Fcn  Expr=u(3)
  " 1" : Outport  VectorParamsAs1DForOutWhenUnconnected=off
  " 2" : Outport  Port=2  VectorParamsAs1DForOutWhenUnconnected=off
  wires:
  f/1 -> Add/1, Product/2
  Product/1 -> Mux1/2, Add/2
  1/1 -> T/1, h/1, f/1
  Add/1 -> Mux/2
  h/1 -> Mux1/3, Mux/3
  T/1 -> Mux1/1, Mux/1
  Mux/1 -> " 1"/1
  Mux1/1 -> " 2"/1
  u122/1 -> Manual Switch/2, Saturation/1
  Saturation/1 -> Manual Switch/1
  Manual Switch/1 -> Product/1

== system Red_problema1_imc_nuevo/Subsystem/inter_E1/bypass1 ==
  note: la corriente 1 es la que se introduce al intercambiador
  note: la corriete 2 es la corriente del byapass
  1 : Inport
  u122 : Inport  Port=2
  Add : Sum  Inputs=+-
  Manual Switch : ManualSwitch  CurrentSetting=0
  Mux : Mux  Inputs=3
  Mux1 : Mux  Inputs=3
  Product : Product
  Saturation : Saturate  UpperLimit=0.999999999  LowerLimit=0
  T : Fcn  Expr=u(1)
  f : Fcn  Expr=u(2)
  h : Fcn  Expr=u(3)
  " 1" : Outport  VectorParamsAs1DForOutWhenUnconnected=off
  " 2" : Outport  Port=2  VectorParamsAs1DForOutWhenUnconnected=off
  wires:
  Mux1/1 -> " 2"/1
  Mux/1 -> " 1"/1
  T/1 -> Mux/1, Mux1/1
  h/1 -> Mux/3, Mux1/3
  Add/1 -> Mux/2
  1/1 -> f/1, h/1, T/1
  Product/1 -> Add/2, Mux1/2
  f/1 -> Product/2, Add/1
  Saturation/1 -> Manual Switch/1
  u122/1 -> Manual Switch/2, Saturation/1
  Manual Switch/1 -> Product/1

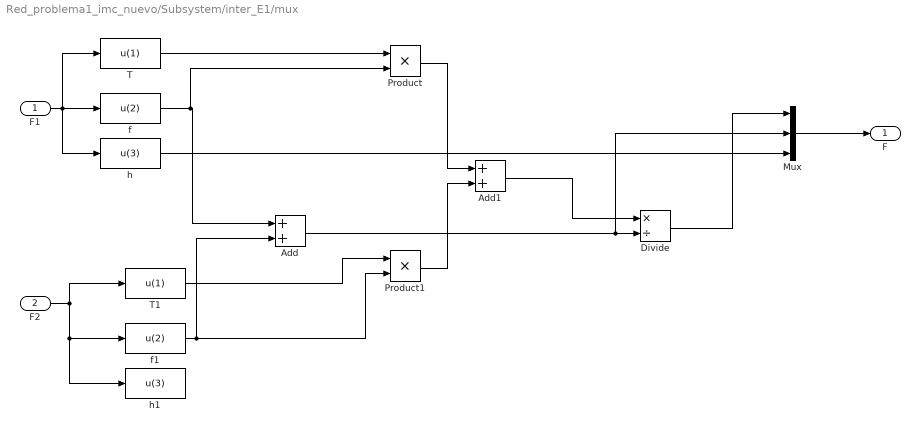
== system Red_problema1_imc_nuevo/Subsystem/inter_E1/mux ==
  F1 : Inport
  F2 : Inport  Port=2
  Add : Sum
  Add1 : Sum
  Divide : Product  Inputs=*/
  Mux : Mux  Inputs=3
  Product : Product
  Product1 : Product
  T : Fcn  Expr=u(1)
  T1 : Fcn  Expr=u(1)
  f : Fcn  Expr=u(2)
  f1 : Fcn  Expr=u(2)
  h : Fcn  Expr=u(3)
  h1 : Fcn  Expr=u(3)
  "F " : Outport  VectorParamsAs1DForOutWhenUnconnected=off
  wires:
  h/1 -> Mux/3
  Divide/1 -> Mux/1
  Add/1 -> Divide/2, Mux/2
  Add1/1 -> Divide/1
  Product1/1 -> Add1/2
  f1/1 -> Product1/2, Add/2
  T1/1 -> Product1/1
  Product/1 -> Add1/1
  T/1 -> Product/1
  F2/1 -> T1/1, f1/1, h1/1
  f/1 -> Add/1, Product/2
  F1/1 -> T/1, h/1, f/1
  Mux/1 -> "F "/1

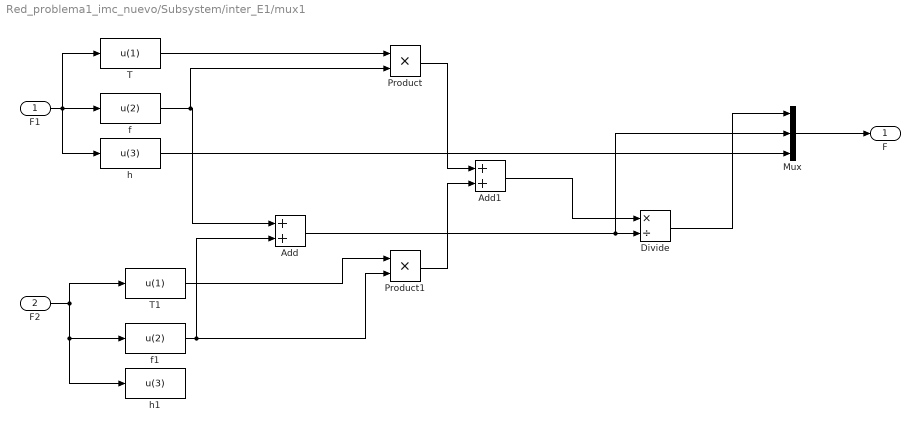
== system Red_problema1_imc_nuevo/Subsystem/inter_E1/mux1 ==
  F1 : Inport
  F2 : Inport  Port=2
  Add : Sum
  Add1 : Sum
  Divide : Product  Inputs=*/
  Mux : Mux  Inputs=3
  Product : Product
  Product1 : Product
  T : Fcn  Expr=u(1)
  T1 : Fcn  Expr=u(1)
  f : Fcn  Expr=u(2)
  f1 : Fcn  Expr=u(2)
  h : Fcn  Expr=u(3)
  h1 : Fcn  Expr=u(3)
  "F " : Outport  VectorParamsAs1DForOutWhenUnconnected=off
  wires:
  Mux/1 -> "F "/1
  F1/1 -> f/1, h/1, T/1
  f/1 -> Product/2, Add/1
  F2/1 -> h1/1, f1/1, T1/1
  T/1 -> Product/1
  Product/1 -> Add1/1
  T1/1 -> Product1/1
  f1/1 -> Add/2, Product1/2
  Product1/1 -> Add1/2
  Add1/1 -> Divide/1
  Add/1 -> Mux/2, Divide/2
  Divide/1 -> Mux/1
  h/1 -> Mux/3

== system Red_problema1_imc_nuevo/Subsystem/inter_E2/bypass ==
  note: la corriente 1 es la que se introduce al intercambiador
  note: la corriete 2 es la corriente del byapass
  1 : Inport
  u122 : Inport  Port=2
  Add : Sum  Inputs=+-
  Manual Switch : ManualSwitch  CurrentSetting=0
  Mux : Mux  Inputs=3
  Mux1 : Mux  Inputs=3
  Product : Product
  Saturation : Saturate  UpperLimit=0.999999999  LowerLimit=0
  T : Fcn  Expr=u(1)
  f : Fcn  Expr=u(2)
  h : Fcn  Expr=u(3)
  " 1" : Outport  VectorParamsAs1DForOutWhenUnconnected=off
  " 2" : Outport  Port=2  VectorParamsAs1DForOutWhenUnconnected=off
  wires:
  Mux1/1 -> " 2"/1
  Mux/1 -> " 1"/1
  T/1 -> Mux/1, Mux1/1
  h/1 -> Mux/3, Mux1/3
  Add/1 -> Mux/2
  1/1 -> f/1, h/1, T/1
  Product/1 -> Add/2, Mux1/2
  f/1 -> Product/2, Add/1
  Saturation/1 -> Manual Switch/1
  u122/1 -> Manual Switch/2, Saturation/1
  Manual Switch/1 -> Product/1

== system Red_problema1_imc_nuevo/Subsystem/inter_E2/bypass1 ==
  note: la corriete 2 es la corriente del byapass
  note: la corriente 1 es la que se introduce al intercambiador
  1 : Inport
  u122 : Inport  Port=2
  Add : Sum  Inputs=+-
  Manual Switch : ManualSwitch  CurrentSetting=0
  Mux : Mux  Inputs=3
  Mux1 : Mux  Inputs=3
  Product : Product
  Saturation : Saturate  UpperLimit=0.999999999  LowerLimit=0
  T : Fcn  Expr=u(1)
  f : Fcn  Expr=u(2)
  h : Fcn  Expr=u(3)
  " 1" : Outport  VectorParamsAs1DForOutWhenUnconnected=off
  " 2" : Outport  Port=2  VectorParamsAs1DForOutWhenUnconnected=off
  wires:
  f/1 -> Add/1, Product/2
  Product/1 -> Mux1/2, Add/2
  1/1 -> T/1, h/1, f/1
  Add/1 -> Mux/2
  h/1 -> Mux1/3, Mux/3
  T/1 -> Mux1/1, Mux/1
  Mux/1 -> " 1"/1
  Mux1/1 -> " 2"/1
  Saturation/1 -> Manual Switch/1
  u122/1 -> Manual Switch/2, Saturation/1
  Manual Switch/1 -> Product/1

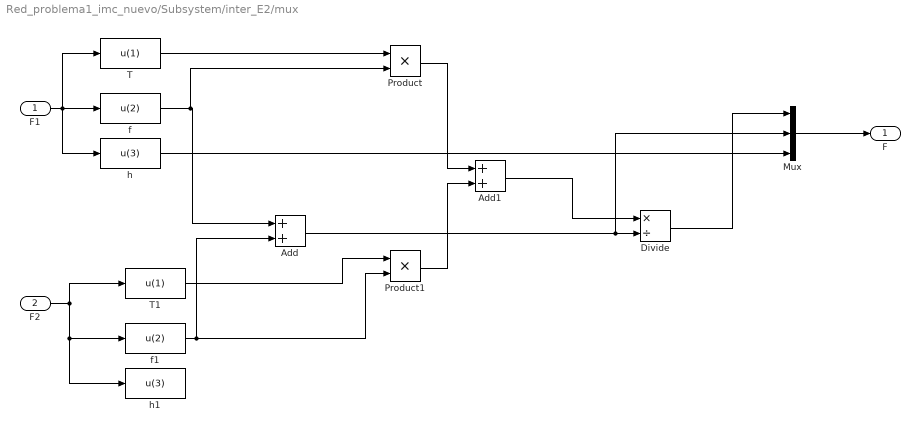
== system Red_problema1_imc_nuevo/Subsystem/inter_E2/mux ==
  F1 : Inport
  F2 : Inport  Port=2
  Add : Sum
  Add1 : Sum
  Divide : Product  Inputs=*/
  Mux : Mux  Inputs=3
  Product : Product
  Product1 : Product
  T : Fcn  Expr=u(1)
  T1 : Fcn  Expr=u(1)
  f : Fcn  Expr=u(2)
  f1 : Fcn  Expr=u(2)
  h : Fcn  Expr=u(3)
  h1 : Fcn  Expr=u(3)
  "F " : Outport  VectorParamsAs1DForOutWhenUnconnected=off
  wires:
  Mux/1 -> "F "/1
  F1/1 -> f/1, h/1, T/1
  f/1 -> Product/2, Add/1
  F2/1 -> h1/1, f1/1, T1/1
  T/1 -> Product/1
  Product/1 -> Add1/1
  T1/1 -> Product1/1
  f1/1 -> Add/2, Product1/2
  Product1/1 -> Add1/2
  Add1/1 -> Divide/1
  Add/1 -> Mux/2, Divide/2
  Divide/1 -> Mux/1
  h/1 -> Mux/3

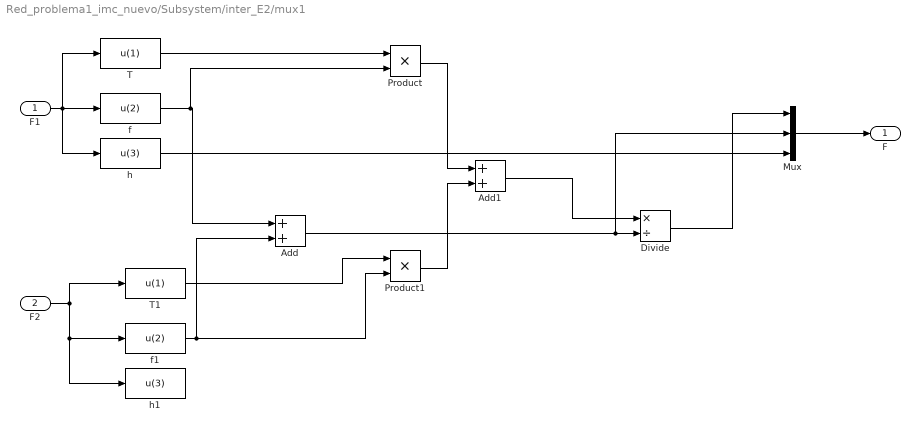
== system Red_problema1_imc_nuevo/Subsystem/inter_E2/mux1 ==
  F1 : Inport
  F2 : Inport  Port=2
  Add : Sum
  Add1 : Sum
  Divide : Product  Inputs=*/
  Mux : Mux  Inputs=3
  Product : Product
  Product1 : Product
  T : Fcn  Expr=u(1)
  T1 : Fcn  Expr=u(1)
  f : Fcn  Expr=u(2)
  f1 : Fcn  Expr=u(2)
  h : Fcn  Expr=u(3)
  h1 : Fcn  Expr=u(3)
  "F " : Outport  VectorParamsAs1DForOutWhenUnconnected=off
  wires:
  h/1 -> Mux/3
  Divide/1 -> Mux/1
  Add/1 -> Divide/2, Mux/2
  Add1/1 -> Divide/1
  Product1/1 -> Add1/2
  f1/1 -> Product1/2, Add/2
  T1/1 -> Product1/1
  Product/1 -> Add1/1
  T/1 -> Product/1
  F2/1 -> T1/1, f1/1, h1/1
  f/1 -> Add/1, Product/2
  F1/1 -> T/1, h/1, f/1
  Mux/1 -> "F "/1

== system Red_problema1_imc_nuevo/Subsystem/inter_E3/bypass ==
  note: la corriete 2 es la corriente del byapass
  note: la corriente 1 es la que se introduce al intercambiador
  1 : Inport
  u122 : Inport  Port=2
  Add : Sum  Inputs=+-
  Manual Switch : ManualSwitch  CurrentSetting=0
  Mux : Mux  Inputs=3
  Mux1 : Mux  Inputs=3
  Product : Product
  Saturation : Saturate  UpperLimit=0.999999999  LowerLimit=0
  T : Fcn  Expr=u(1)
  f : Fcn  Expr=u(2)
  h : Fcn  Expr=u(3)
  " 1" : Outport  VectorParamsAs1DForOutWhenUnconnected=off
  " 2" : Outport  Port=2  VectorParamsAs1DForOutWhenUnconnected=off
  wires:
  f/1 -> Add/1, Product/2
  Product/1 -> Mux1/2, Add/2
  1/1 -> T/1, h/1, f/1
  Add/1 -> Mux/2
  h/1 -> Mux1/3, Mux/3
  T/1 -> Mux1/1, Mux/1
  Mux/1 -> " 1"/1
  Mux1/1 -> " 2"/1
  Saturation/1 -> Manual Switch/1
  u122/1 -> Manual Switch/2, Saturation/1
  Manual Switch/1 -> Product/1

== system Red_problema1_imc_nuevo/Subsystem/inter_E3/bypass1 ==
  note: la corriente 1 es la que se introduce al intercambiador
  note: la corriete 2 es la corriente del byapass
  1 : Inport
  u122 : Inport  Port=2
  Add : Sum  Inputs=+-
  Manual Switch : ManualSwitch  CurrentSetting=0
  Mux : Mux  Inputs=3
  Mux1 : Mux  Inputs=3
  Product : Product
  Saturation : Saturate  UpperLimit=0.999999999  LowerLimit=0
  T : Fcn  Expr=u(1)
  f : Fcn  Expr=u(2)
  h : Fcn  Expr=u(3)
  " 1" : Outport  VectorParamsAs1DForOutWhenUnconnected=off
  " 2" : Outport  Port=2  VectorParamsAs1DForOutWhenUnconnected=off
  wires:
  Mux1/1 -> " 2"/1
  Mux/1 -> " 1"/1
  T/1 -> Mux/1, Mux1/1
  h/1 -> Mux/3, Mux1/3
  Add/1 -> Mux/2
  1/1 -> f/1, h/1, T/1
  Product/1 -> Add/2, Mux1/2
  f/1 -> Product/2, Add/1
  Saturation/1 -> Manual Switch/1
  u122/1 -> Manual Switch/2, Saturation/1
  Manual Switch/1 -> Product/1

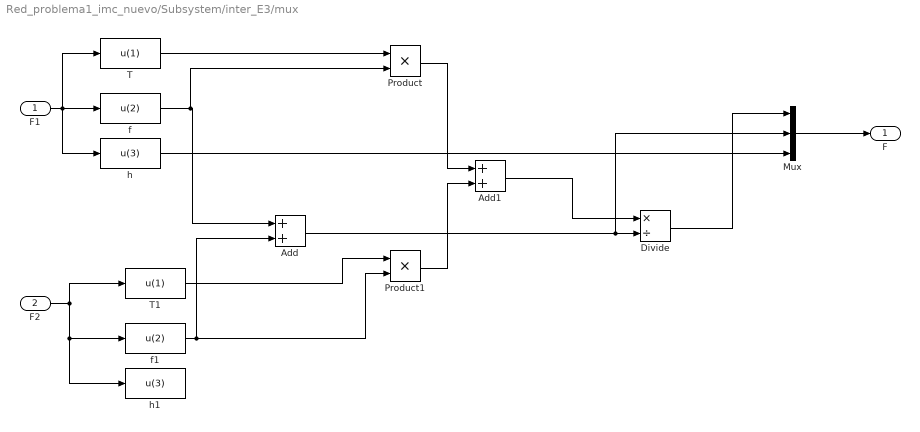
== system Red_problema1_imc_nuevo/Subsystem/inter_E3/mux ==
  F1 : Inport
  F2 : Inport  Port=2
  Add : Sum
  Add1 : Sum
  Divide : Product  Inputs=*/
  Mux : Mux  Inputs=3
  Product : Product
  Product1 : Product
  T : Fcn  Expr=u(1)
  T1 : Fcn  Expr=u(1)
  f : Fcn  Expr=u(2)
  f1 : Fcn  Expr=u(2)
  h : Fcn  Expr=u(3)
  h1 : Fcn  Expr=u(3)
  "F " : Outport  VectorParamsAs1DForOutWhenUnconnected=off
  wires:
  h/1 -> Mux/3
  Divide/1 -> Mux/1
  Add/1 -> Divide/2, Mux/2
  Add1/1 -> Divide/1
  Product1/1 -> Add1/2
  f1/1 -> Product1/2, Add/2
  T1/1 -> Product1/1
  Product/1 -> Add1/1
  T/1 -> Product/1
  F2/1 -> T1/1, f1/1, h1/1
  f/1 -> Add/1, Product/2
  F1/1 -> T/1, h/1, f/1
  Mux/1 -> "F "/1

== system Red_problema1_imc_nuevo/Subsystem/inter_E3/mux1 ==
  F1 : Inport
  F2 : Inport  Port=2
  Add : Sum
  Add1 : Sum
  Divide : Product  Inputs=*/
  Mux : Mux  Inputs=3
  Product : Product
  Product1 : Product
  T : Fcn  Expr=u(1)
  T1 : Fcn  Expr=u(1)
  f : Fcn  Expr=u(2)
  f1 : Fcn  Expr=u(2)
  h : Fcn  Expr=u(3)
  h1 : Fcn  Expr=u(3)
  "F " : Outport  VectorParamsAs1DForOutWhenUnconnected=off
  wires:
  Mux/1 -> "F "/1
  F1/1 -> f/1, h/1, T/1
  f/1 -> Product/2, Add/1
  F2/1 -> h1/1, f1/1, T1/1
  T/1 -> Product/1
  Product/1 -> Add1/1
  T1/1 -> Product1/1
  f1/1 -> Add/2, Product1/2
  Product1/1 -> Add1/2
  Add1/1 -> Divide/1
  Add/1 -> Mux/2, Divide/2
  Divide/1 -> Mux/1
  h/1 -> Mux/3

== system Red_problema1_imc_nuevo/Subsystem/inter_Ecu/bypass ==
  note: la corriente 1 es la que se introduce al intercambiador
  note: la corriete 2 es la corriente del byapass
  1 : Inport
  u122 : Inport  Port=2
  Add : Sum  Inputs=+-
  Manual Switch : ManualSwitch  CurrentSetting=0
  Mux : Mux  Inputs=3
  Mux1 : Mux  Inputs=3
  Product : Product
  Saturation : Saturate  UpperLimit=0.999999999  LowerLimit=0
  T : Fcn  Expr=u(1)
  f : Fcn  Expr=u(2)
  h : Fcn  Expr=u(3)
  " 1" : Outport  VectorParamsAs1DForOutWhenUnconnected=off
  " 2" : Outport  Port=2  VectorParamsAs1DForOutWhenUnconnected=off
  wires:
  Mux1/1 -> " 2"/1
  Mux/1 -> " 1"/1
  T/1 -> Mux/1, Mux1/1
  h/1 -> Mux/3, Mux1/3
  Add/1 -> Mux/2
  1/1 -> f/1, h/1, T/1
  Product/1 -> Add/2, Mux1/2
  f/1 -> Product/2, Add/1
  Saturation/1 -> Manual Switch/1
  u122/1 -> Manual Switch/2, Saturation/1
  Manual Switch/1 -> Product/1

== system Red_problema1_imc_nuevo/Subsystem/inter_Ecu/bypass1 ==
  note: la corriete 2 es la corriente del byapass
  note: la corriente 1 es la que se introduce al intercambiador
  1 : Inport
  u122 : Inport  Port=2
  Add : Sum  Inputs=+-
  Manual Switch : ManualSwitch  CurrentSetting=0
  Mux : Mux  Inputs=3
  Mux1 : Mux  Inputs=3
  Product : Product
  Saturation : Saturate  UpperLimit=0.999999999  LowerLimit=0
  Scope : Scope
  T : Fcn  Expr=u(1)
  f : Fcn  Expr=u(2)
  h : Fcn  Expr=u(3)
  " 1" : Outport  VectorParamsAs1DForOutWhenUnconnected=off
  " 2" : Outport  Port=2  VectorParamsAs1DForOutWhenUnconnected=off
  wires:
  f/1 -> Add/1, Product/2
  Product/1 -> Scope/1, Mux1/2, Add/2
  1/1 -> T/1, h/1, f/1
  Add/1 -> Mux/2
  h/1 -> Mux1/3, Mux/3
  T/1 -> Mux1/1, Mux/1
  Mux/1 -> " 1"/1
  Mux1/1 -> " 2"/1
  Saturation/1 -> Manual Switch/1
  u122/1 -> Manual Switch/2, Saturation/1
  Manual Switch/1 -> Product/1

== system Red_problema1_imc_nuevo/Subsystem/inter_Ecu/mux ==
  F1 : Inport
  F2 : Inport  Port=2
  Add : Sum
  Add1 : Sum
  Divide : Product  Inputs=*/
  Mux : Mux  Inputs=3
  Product : Product
  Product1 : Product
  T : Fcn  Expr=u(1)
  T1 : Fcn  Expr=u(1)
  f : Fcn  Expr=u(2)
  f1 : Fcn  Expr=u(2)
  h : Fcn  Expr=u(3)
  h1 : Fcn  Expr=u(3)
  "F " : Outport  VectorParamsAs1DForOutWhenUnconnected=off
  wires:
  Mux/1 -> "F "/1
  F1/1 -> f/1, h/1, T/1
  f/1 -> Product/2, Add/1
  F2/1 -> h1/1, f1/1, T1/1
  T/1 -> Product/1
  Product/1 -> Add1/1
  T1/1 -> Product1/1
  f1/1 -> Add/2, Product1/2
  Product1/1 -> Add1/2
  Add1/1 -> Divide/1
  Add/1 -> Mux/2, Divide/2
  Divide/1 -> Mux/1
  h/1 -> Mux/3

== system Red_problema1_imc_nuevo/Subsystem/inter_Ecu/mux1 ==
  F1 : Inport
  F2 : Inport  Port=2
  Add : Sum
  Add1 : Sum
  Divide : Product  Inputs=*/
  Mux : Mux  Inputs=3
  Product : Product
  Product1 : Product
  T : Fcn  Expr=u(1)
  T1 : Fcn  Expr=u(1)
  f : Fcn  Expr=u(2)
  f1 : Fcn  Expr=u(2)
  h : Fcn  Expr=u(3)
  h1 : Fcn  Expr=u(3)
  "F " : Outport  VectorParamsAs1DForOutWhenUnconnected=off
  wires:
  h/1 -> Mux/3
  Divide/1 -> Mux/1
  Add/1 -> Divide/2, Mux/2
  Add1/1 -> Divide/1
  Product1/1 -> Add1/2
  f1/1 -> Product1/2, Add/2
  T1/1 -> Product1/1
  Product/1 -> Add1/1
  T/1 -> Product/1
  F2/1 -> T1/1, f1/1, h1/1
  f/1 -> Add/1, Product/2
  F1/1 -> T/1, h/1, f/1
  Mux/1 -> "F "/1
